simulink model "HangingPendulum"  (R2012b)
settings: Solver=ode45  StartTime=0.0  StopTime=10.0  RelTol=1e-3
values from neighbouring files (symbols this model uses):
  b = 0    [runPendulum.m]
  Final_value = 0    [runPendulum.m]
  g = 10    [runPendulum.m]
  Initial_value = 0    [runPendulum.m]
  J = Jc+m*lc^2    (= 1)    [runPendulum.m]
  lc = 1    [runPendulum.m]
  m = 1    [runPendulum.m]
  Sample_time = 0    [runPendulum.m]
  Step_time = 1    [runPendulum.m]
settings Model: Creator=cat  LastModifiedBy=cat
settings DataIOCC: LoadInitialState=on

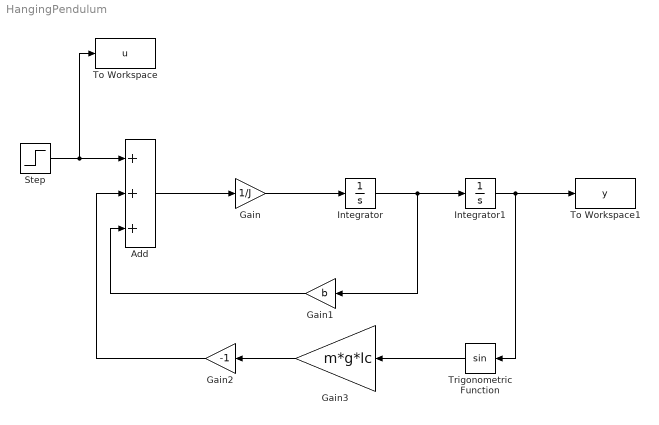
== system HangingPendulum ==
  Add : Sum  Inputs=+++
  Gain : Gain  Gain=1/J
  Gain1 : Gain  Gain=b
  Gain2 : Gain  Gain=-1
  Gain3 : Gain  Gain=m*g*lc
  Integrator : Integrator
  Integrator1 : Integrator
  Step : Step  Time=Step_time  Before=Initial_value  After=Final_value  SampleTime=Sample_time
  To Workspace : ToWorkspace  VariableName=u  SampleTime=-1
  To Workspace1 : ToWorkspace  VariableName=y  SampleTime=-1
  Trigonometric Function : Trigonometry
  wires:
  Step/1 -> To Workspace/1, Add/1
  Add/1 -> Gain/1
  Gain/1 -> Integrator/1
  Integrator/1 -> Gain1/1, Integrator1/1
  Gain1/1 -> Add/3
  Trigonometric Function/1 -> Gain3/1
  Gain3/1 -> Gain2/1
  Gain2/1 -> Add/2
  Integrator1/1 -> To Workspace1/1, Trigonometric Function/1
